simulink model "LAB3_Euler_eq"  (R2022b)
settings: Solver=ode4  StartTime=0.0  StopTime=100  FixedStep=0.1  RelTol=1e-3
values from neighbouring files (symbols this model uses):
  euler_angles_0 = [1;1;1]    [LAB_03.m]
  I = diag([0.025 , 0.055 , 0.07])    [LAB_03.m]
  w0 = [2*pi , 1 , 0.1]    [LAB_03.m]
libraries: matrix_library x1
settings Model: Creator=ludov  LastModifiedBy=ludov

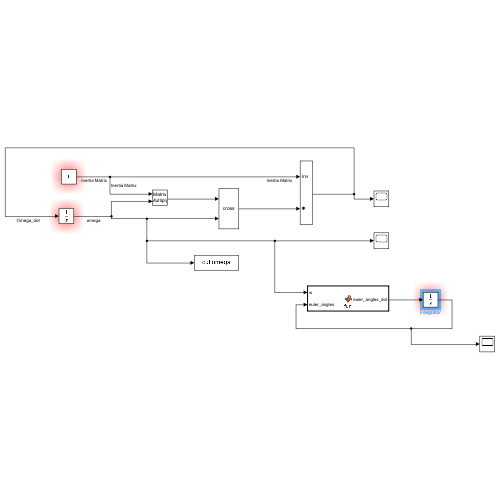
[thumbnail: Simulink's stored preview of the top-level diagram]
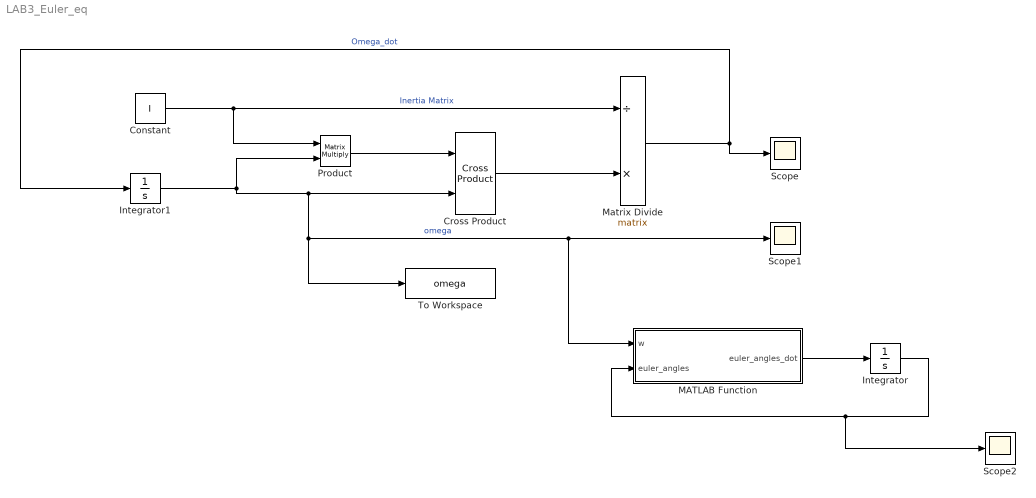
== system LAB3_Euler_eq ==
  Constant : Constant  Value=I
  Cross Product : matrix_library/Cross Product
  Integrator : Integrator  InitialCondition=euler_angles_0
  Integrator1 : Integrator  InitialCondition=w0
  MATLAB Function : MATLAB Function  TreatAsAtomicUnit=on
  Matrix Divide : Product  Inputs=/*  Multiplication=Matrix(*)
  Product : Product  Multiplication=Matrix(*)
  Scope : Scope
  Scope1 : Scope
  Scope2 : Scope
  To Workspace : ToWorkspace  VariableName=omega  SaveFormat=Timeseries  SampleTime=-1
  wires:
  Integrator1/1 -> To Workspace/1, MATLAB Function/1(w), Scope1/1, Cross Product/2, Product/2  "omega"
  Constant/1 -> Product/1, Matrix Divide/1  "Inertia Matrix"
  Product/1 -> Cross Product/1
  Cross Product/1 -> Matrix Divide/2
  Matrix Divide/1 -> Integrator1/1, Scope/1  "Omega_dot"
  MATLAB Function/1(euler_angles_dot) -> Integrator/1
  Integrator/1 -> Scope2/1, MATLAB Function/2(euler_angles)

== matlab function LAB3_Euler_eq/MATLAB Function ==
  data: w input; euler_angles_dot output; euler_angles input
function euler_angles_dot = fun(w, euler_angles)
    
    % Define data
    phi         = euler_angles(1);
    theta       = euler_angles(2);
    psi         = euler_angles(3);

%Calculate derivatives of Euler's angles
    phi_dot     = (w(1)*sin(psi) + w(2)*cos(psi))/sin(theta);
    theta_dot   = w(1)*cos(psi) - w(2)*sin(psi);
    psi_dot     = w(3) - (w(1)*sin(psi) + w(1)*cos(psi)) * (cos(theta_dot)/sin(theta));

    euler_angles_dot=[phi_dot;theta_dot;psi_dot];


y = u;
